simulink model "circuitTestSimulink_MDKTemplate_3DElectrical_Exp_Short"  (R2024b)
settings: Solver=VariableStepAuto  StartTime=0.0  StopTime=1.5e-6  FixedStep=1e-12  MaxStep=1e-11  MinStep=1e-23  RelTol=1  AbsTol=1
undefined symbols (not defined in the file or in its folder): FMIKit
libraries: fl_lib x15, nesl_utility x11, ee_lib x2
settings Model: Creator=ezzbj2  LastModifiedBy=Bawar
settings SolverCC: AutoScaleAbsTol=off  InitialStep=1e-11  MaxOrder=2  MaxConsecutiveMinStep=20  AllowMultiTaskInputOutput=on  ShapePreserveControl=EnableAll  ZeroCrossControl=DisableAll  SolverResetMethod=Robust  PositivePriorityOrder=on
settings RTWCC: GPUComputeCapability=3.5

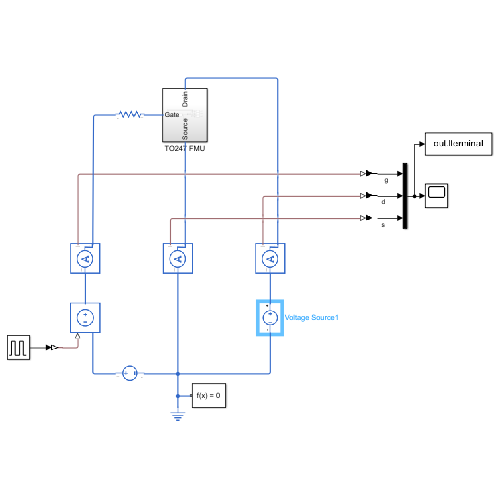
[thumbnail: Simulink's stored preview of the top-level diagram]
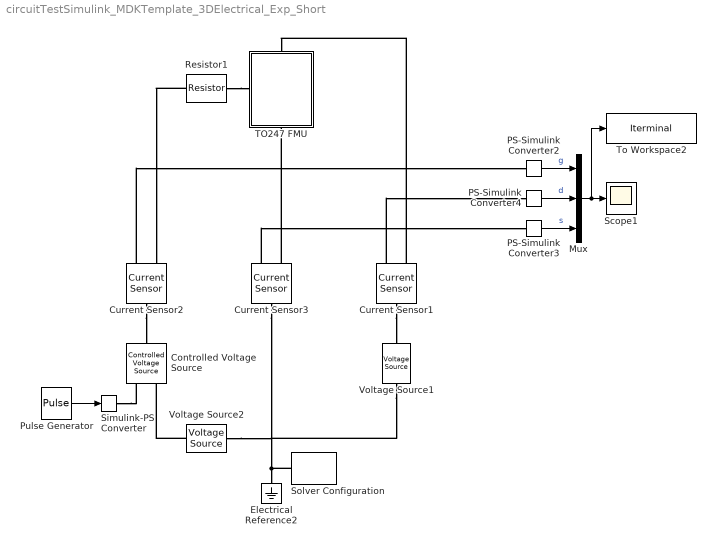
== system circuitTestSimulink_MDKTemplate_3DElectrical_Exp_Short ==
  Controlled Voltage Source : fl_lib/Electrical/Electrical Sources/Controlled Voltage Source
  Current Sensor1 : fl_lib/Electrical/Electrical Sensors/Current Sensor
  Current Sensor2 : fl_lib/Electrical/Electrical Sensors/Current Sensor
  Current Sensor3 : fl_lib/Electrical/Electrical Sensors/Current Sensor
  Electrical Reference2 : fl_lib/Electrical/Electrical Elements/Electrical Reference
  Mux : Mux  Inputs=3
  PS-Simulink Converter2 : nesl_utility/PS-Simulink Converter  PhysicalDomain=network_engine_domain  SubClassName=ps_output  LeftPortType=input  RightPortType=output  PseudoPeriodic=off  Frequencies=[]  VectorFormat=inherit  Unit=inherit  AffineConversion=off
  PS-Simulink Converter3 : nesl_utility/PS-Simulink Converter  PhysicalDomain=network_engine_domain  SubClassName=ps_output  LeftPortType=input  RightPortType=output  PseudoPeriodic=off  Frequencies=[]  VectorFormat=inherit  Unit=inherit  AffineConversion=off
  PS-Simulink Converter4 : nesl_utility/PS-Simulink Converter  PhysicalDomain=network_engine_domain  SubClassName=ps_output  LeftPortType=input  RightPortType=output  PseudoPeriodic=off  Frequencies=[]  VectorFormat=inherit  Unit=inherit  AffineConversion=off
  Pulse Generator : DiscretePulseGenerator  PulseType=Time based  Amplitude=20  Period=1e-6  PulseWidth=50
  Resistor1 : fl_lib/Electrical/Electrical Elements/Resistor  R=2 Ohm  i_specify=off  i_priority=None  i=0 A  i_nominal_specify=off  i_nominal_value=1  i_nominal_unit=A  v_specify=off  v_priority=None  v=0 V  v_nominal_specify=off  v_nominal_value=1  v_nominal_unit=V
  Scope1 : Scope
  Simulink-PS Converter : nesl_utility/Simulink-PS Converter  PhysicalDomain=network_engine_domain  SubClassName=ps_input  LeftPortType=input  RightPortType=output  PseudoPeriodic=off  Frequencies=[]  NoiseDistribution=none  NoiseParameters=[]  Unit=1  AffineConversion=off  FilteringAndDerivatives=provide  SimscapeFilterOrder=1  InputFilterTimeConstant=0.001  UdotUserProvided=0
  Solver Configuration : nesl_utility/Solver Configuration  PhysicalDomain=network_engine_domain  SubClassName=solver  LeftPortType=input  RightPortType=generic  Tones=[]  Harmonics=[]  SimulateNoise=off  Profile=off  UseLocalSampling=off  EnableSwitchedLinearOptims=on  FrequencyDomain=off  UseCCode=off  RelTol=0.001  AbsTol=0.001  MinStep=1e-09  ToWorkspace=off  RevertToSquareIcSolve=off  NumHomotopyIterations=100  PhasorMode=off  PhasorModeNumHarmonics=1  ConsistencySolver=NEWTON_XTOL_AFTER_FTOL  IndexReductionMethod=None  DoDC=off  ResidualTolerance=1e-09  ConsistencyTolSource=GLOBAL  ConsistencyAbsTol=0.01  ConsistencyRelTol=0.001  ConsistencyTolFactor=0.1  UseLocalSolver=off  LocalSolverChoice=NE_BACKWARD_EULER_ADVANCER  ResolveIndetEquations=on  FunctionEvalNumThread=1  LocalSolverSampleTime=1e-12  DoFixedCost=off  MaxNonlinIter=30  MaxModeIter=2  ComputeImpulses=on  ImpulseIterations=2  LinearAlgebra=auto  LinearAlgebraNumThread=0  EquationFormulation=NE_TIME_EF  DelaysMemoryBudget=1024  AutomaticFiltering=off  FilteringTimeConstant=0.001  PartitionStorageMethod=EXHAUSTIVE  PartitionMemoryBudget=1024  PartitionMethod=ROBUST  MultibodyUseLocalSolver=off  MultibodyLocalSolverChoice=ODE1  MultibodyLocalSolverSampleTime=0.001
  TO247 FMU : Subsystem
      settings: PortSchema="{\"entries\":[{\"content\":{\"sides\":[{\"content\":{\"connectorIds\":[\"LConn1\"]},\"type\":\"ConnectorPlacement.EquallySpacedRectSide\",\"uuid\":\"1a7c621a-b2c4-44d6-8085-8acdfe65af3e\"},{\"content\":{\"side\":\"RIGHT\"},\"type\":\"ConnectorPlacement.EquallySpacedRectSide\",\"uuid\":\"009b5a79-97ab-42cc-83a0-e109b769c9f7\"},{\"content\":{\"connectorIds\":[\"LConn2\"],\"side\":\"TOP\"},\"type\":\"ConnectorPlacement.EquallySpacedRectSide\",\"uuid\":\"b2698f3e-d975-41db-922f-800e4c377170\"},{\"content\":{\"connectorIds\":[\"RConn1\"],\"side\":\"BOTTOM\"},\"type\":\"ConnectorPlacement.EquallySpacedRectSide\",\"uuid\":\"c87b7d4f-b69b-4cab-ae10-03d23c792008\"}]},\"type\":\"ConnectorPlacement.EquallySpacedConnector\",\"uuid\":\"776127ee-5564-4d8f-a192-88fd759918ca\"}],\"packageUris\":[\"http://schema.mathworks.com/mf0/Connector/R2020b\"],\"version\":\"1.0\"}"
  To Workspace2 : ToWorkspace  VariableName=Iterminal  SaveFormat=Timeseries  SampleTime=-1
  Voltage Source1 : ee_lib/Sources/Voltage Source  dc_voltage=400 V  ac_voltage=0 V  ac_shift=0 rad  ac_frequency=60 Hz  noise_mode=ee.enum.sources.noise.Disabled  PSD=0 V^2/Hz  sample_time=1e-3 s  repeatability=ee.enum.sources.repeatability.NotRepeatable  user_seed=0  auto_seed=545404223  i_specify=off  i_priority=None  i=0 A  i_nominal_specify=off  i_nominal_value=1  i_nominal_unit=A  v_specify=off  v_priority=None  v=0 V  v_nominal_specify=off  v_nominal_value=1  v_nominal_unit=V
  Voltage Source2 : ee_lib/Sources/Voltage Source  dc_voltage=-5 V  ac_voltage=0 V  ac_shift=0 rad  ac_frequency=60 Hz  noise_mode=ee.enum.sources.noise.Disabled  PSD=0 V^2/Hz  sample_time=1e-3 s  repeatability=ee.enum.sources.repeatability.NotRepeatable  user_seed=0  auto_seed=3499211588  i_specify=off  i_priority=None  i=0 A  i_nominal_specify=off  i_nominal_value=1  i_nominal_unit=A  v_specify=off  v_priority=None  v=0 V  v_nominal_specify=off  v_nominal_value=1  v_nominal_unit=V
  wires:
  Mux/1 -> Scope1/1, To Workspace2/1
  PS-Simulink Converter2/1 -> Mux/1  "g"
  PS-Simulink Converter3/1 -> Mux/3  "s"
  PS-Simulink Converter4/1 -> Mux/2  "d"
  Pulse Generator/1 -> Simulink-PS Converter/1
  connections:
  Current Sensor2/RConn1 -- PS-Simulink Converter2/LConn1
  Current Sensor3/RConn1 -- PS-Simulink Converter3/LConn1
  Current Sensor1/RConn1 -- PS-Simulink Converter4/LConn1
  Current Sensor1/LConn1 -- Voltage Source1/LConn1
  Current Sensor2/LConn1 -- Controlled Voltage Source/LConn1
  Current Sensor3/RConn2 -- TO247 FMU/RConn1
  Solver Configuration/RConn1 -- Current Sensor3/LConn1 -- Voltage Source1/RConn1 -- Voltage Source2/RConn1 -- Electrical Reference2/LConn1
  Resistor1/LConn1 -- TO247 FMU/LConn1
  Current Sensor1/RConn2 -- TO247 FMU/LConn2
  Simulink-PS Converter/RConn1 -- Controlled Voltage Source/RConn1
  Voltage Source2/LConn1 -- Controlled Voltage Source/RConn2
  Resistor1/RConn1 -- Current Sensor2/RConn2

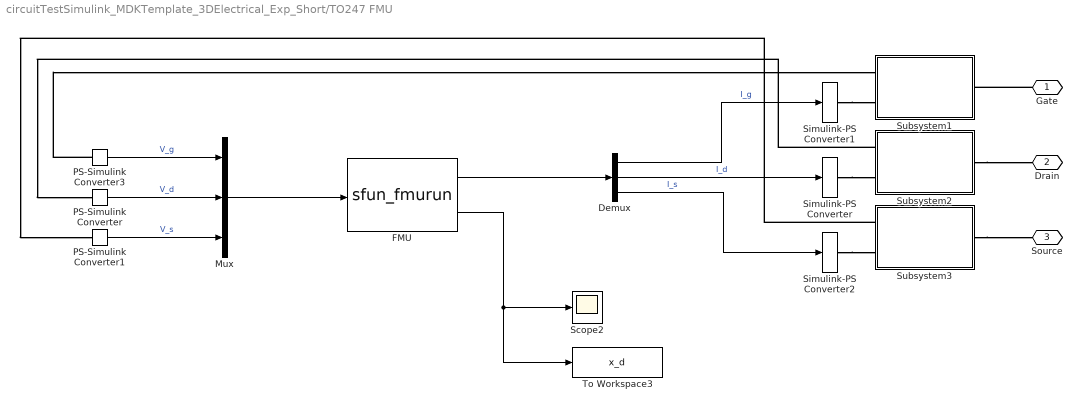
== system circuitTestSimulink_MDKTemplate_3DElectrical_Exp_Short/TO247 FMU ==
  Demux : Demux  Outputs=3
  FMU : S-Function  LoadFcn=FMIKit.setSFunctionParameters(gcb)  FunctionName=sfun_fmurun  Parameters=3.0 0 '{D773325B-AB94-4630-BF85-643EB24FCB80}' 'MDKCircuit_3DElectrical_Exp_Short' FMIKit.getUnzipDirectory(gcb) 0 0 0 '' FMIKit.getSolverRelativeTolerance(bdroot(gcb)) -1 0 10 0 0 [3] [1.0] [2] [9] [3 10] [2 2] [10 11]  SFunctionDeploymentMode=off  EnableBusSupport=off
      settings: DeleteFcn=FMIKit.closeBlockDialog(gcbh)  ModelCloseFcn=FMIKit.closeBlockDialog(gcbh)  DestroyFcn=FMIKit.closeBlockDialog(gcbh)  OpenFcn=FMIKit.showBlockDialog(gcbh);  CloseFcn=FMIKit.closeBlockDialog(gcbh)  ParentCloseFcn=FMIKit.closeBlockDialog(gcbh)
      mask Help: eval('FMIKit.showBlockDialogHelp();')
      mask Display:
      | port_label('input', 1, 'u');
      | port_label('output', 1, 'y');
      | port_label('output', 2, 'x_d');
  Mux : Mux  Inputs=3
  PS-Simulink Converter : nesl_utility/PS-Simulink Converter  PhysicalDomain=network_engine_domain  SubClassName=ps_output  LeftPortType=input  RightPortType=output  PseudoPeriodic=off  Frequencies=[]  VectorFormat=inherit  Unit=inherit  AffineConversion=on
  PS-Simulink Converter1 : nesl_utility/PS-Simulink Converter  PhysicalDomain=network_engine_domain  SubClassName=ps_output  LeftPortType=input  RightPortType=output  PseudoPeriodic=off  Frequencies=[]  VectorFormat=inherit  Unit=inherit  AffineConversion=on
  PS-Simulink Converter3 : nesl_utility/PS-Simulink Converter  PhysicalDomain=network_engine_domain  SubClassName=ps_output  LeftPortType=input  RightPortType=output  PseudoPeriodic=off  Frequencies=[]  VectorFormat=inherit  Unit=inherit  AffineConversion=off
  Scope2 : Scope
  Simulink-PS Converter : nesl_utility/Simulink-PS Converter  PhysicalDomain=network_engine_domain  SubClassName=ps_input  LeftPortType=input  RightPortType=output  PseudoPeriodic=off  Frequencies=[]  NoiseDistribution=none  NoiseParameters=[]  Unit=1  AffineConversion=off  FilteringAndDerivatives=zero  SimscapeFilterOrder=1  InputFilterTimeConstant=1e-11  UdotUserProvided=0
  Simulink-PS Converter1 : nesl_utility/Simulink-PS Converter  PhysicalDomain=network_engine_domain  SubClassName=ps_input  LeftPortType=input  RightPortType=output  PseudoPeriodic=off  Frequencies=[]  NoiseDistribution=none  NoiseParameters=[]  Unit=1  AffineConversion=off  FilteringAndDerivatives=zero  SimscapeFilterOrder=1  InputFilterTimeConstant=1e-11  UdotUserProvided=0
  Simulink-PS Converter2 : nesl_utility/Simulink-PS Converter  PhysicalDomain=network_engine_domain  SubClassName=ps_input  LeftPortType=input  RightPortType=output  PseudoPeriodic=off  Frequencies=[]  NoiseDistribution=none  NoiseParameters=[]  Unit=1  AffineConversion=off  FilteringAndDerivatives=zero  SimscapeFilterOrder=1  InputFilterTimeConstant=1e-11  UdotUserProvided=0
  Subsystem1 : Subsystem
  Subsystem2 : Subsystem
  Subsystem3 : Subsystem
  To Workspace3 : ToWorkspace  VariableName=x_d  SaveFormat=Timeseries  SampleTime=-1
  Gate : PMIOPort  Side=Left
  Drain : PMIOPort  Port=2  Side=Left
  Source : PMIOPort  Port=3  Side=Right
  wires:
  PS-Simulink Converter1/1 -> Mux/3  "V_s"
  PS-Simulink Converter/1 -> Mux/2  "V_d"
  PS-Simulink Converter3/1 -> Mux/1  "V_g"
  Demux/1 -> Simulink-PS Converter1/1  "I_g"
  Demux/2 -> Simulink-PS Converter/1  "I_d"
  Demux/3 -> Simulink-PS Converter2/1  "I_s"
  FMU/1 -> Demux/1
  Mux/1 -> FMU/1
  FMU/2 -> To Workspace3/1, Scope2/1
  connections:
  Subsystem2/LConn1 -- PS-Simulink Converter/LConn1
  PS-Simulink Converter3/LConn1 -- Subsystem1/LConn1
  Subsystem3/LConn1 -- PS-Simulink Converter1/LConn1
  Gate/RConn1 -- Subsystem1/RConn1
  Subsystem2/RConn1 -- Drain/RConn1
  Subsystem3/RConn1 -- Source/RConn1
  Simulink-PS Converter1/RConn1 -- Subsystem1/LConn2
  Simulink-PS Converter/RConn1 -- Subsystem2/LConn2
  Simulink-PS Converter2/RConn1 -- Subsystem3/LConn2

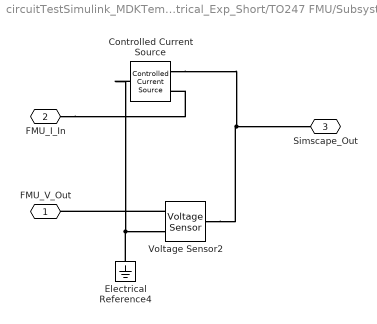
== system circuitTestSimulink_MDKTemplate_3DElectrical_Exp_Short/TO247 FMU/Subsystem1 ==
  Controlled Current Source : fl_lib/Electrical/Electrical Sources/Controlled Current Source
  Electrical Reference4 : fl_lib/Electrical/Electrical Elements/Electrical Reference
  Voltage Sensor2 : fl_lib/Electrical/Electrical Sensors/Voltage Sensor
  FMU_V_Out : PMIOPort  Side=Left
  FMU_I_In : PMIOPort  Port=2  Side=Left
  Simscape_Out : PMIOPort  Port=3  Side=Right
  connections:
  Voltage Sensor2/RConn1 -- FMU_V_Out/RConn1
  FMU_I_In/RConn1 -- Controlled Current Source/RConn1
  Electrical Reference4/LConn1 -- Controlled Current Source/LConn1 -- Voltage Sensor2/RConn2
  Voltage Sensor2/LConn1 -- Controlled Current Source/RConn2 -- Simscape_Out/RConn1

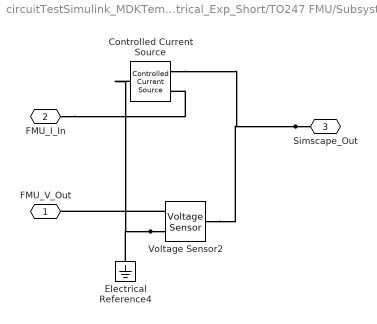
== system circuitTestSimulink_MDKTemplate_3DElectrical_Exp_Short/TO247 FMU/Subsystem2 ==
  Controlled Current Source : fl_lib/Electrical/Electrical Sources/Controlled Current Source
  Electrical Reference4 : fl_lib/Electrical/Electrical Elements/Electrical Reference
  Voltage Sensor2 : fl_lib/Electrical/Electrical Sensors/Voltage Sensor
  FMU_V_Out : PMIOPort  Side=Left
  FMU_I_In : PMIOPort  Port=2  Side=Left
  Simscape_Out : PMIOPort  Port=3  Side=Right
  connections:
  Voltage Sensor2/RConn1 -- FMU_V_Out/RConn1
  FMU_I_In/RConn1 -- Controlled Current Source/RConn1
  Voltage Sensor2/RConn2 -- Electrical Reference4/LConn1 -- Controlled Current Source/LConn1
  Simscape_Out/RConn1 -- Voltage Sensor2/LConn1 -- Controlled Current Source/RConn2

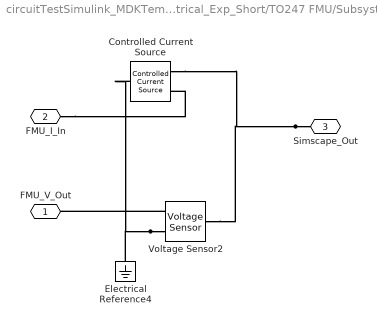
== system circuitTestSimulink_MDKTemplate_3DElectrical_Exp_Short/TO247 FMU/Subsystem3 ==
  Controlled Current Source : fl_lib/Electrical/Electrical Sources/Controlled Current Source
  Electrical Reference4 : fl_lib/Electrical/Electrical Elements/Electrical Reference
  Voltage Sensor2 : fl_lib/Electrical/Electrical Sensors/Voltage Sensor
  FMU_V_Out : PMIOPort  Side=Left
  FMU_I_In : PMIOPort  Port=2  Side=Left
  Simscape_Out : PMIOPort  Port=3  Side=Right
  connections:
  Voltage Sensor2/RConn1 -- FMU_V_Out/RConn1
  FMU_I_In/RConn1 -- Controlled Current Source/RConn1
  Voltage Sensor2/RConn2 -- Electrical Reference4/LConn1 -- Controlled Current Source/LConn1
  Simscape_Out/RConn1 -- Voltage Sensor2/LConn1 -- Controlled Current Source/RConn2
